simulink model "step1"  (R2026a)
settings: Solver=VariableStepAuto
undefined symbols (not defined in the file): F_drive, m
settings Model: Creator=manoj  LastModifiedBy=manoj

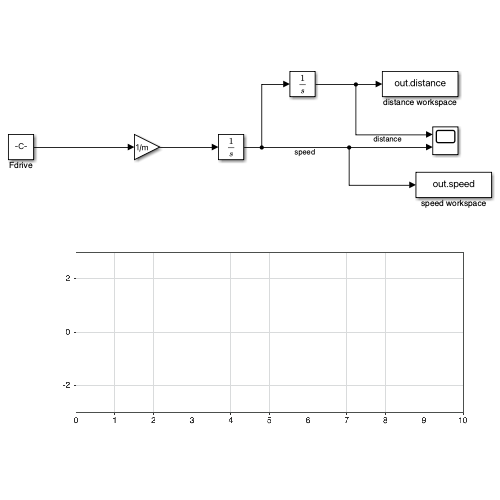
[thumbnail: Simulink's stored preview of the top-level diagram]
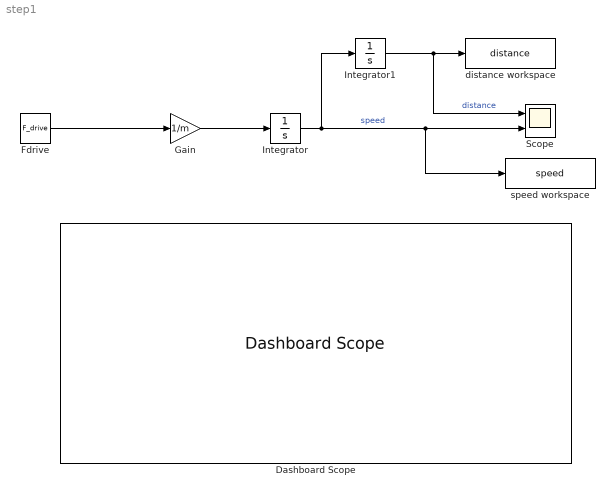
== system step1 ==
  Dashboard Scope : DashboardScope  FontColor=[0.0, 0.0, 0.0]
  Fdrive : Constant  Value=F_drive
  Gain : Gain  Gain=1/m
  Integrator : Integrator
  Integrator1 : Integrator
  Scope : Scope  NumInputPorts=2
      settings: ActiveDisplayYMinimum=-1  ActiveDisplayYMaximum=1
  distance workspace : ToWorkspace  VariableName=distance  SaveFormat=Structure With Time  SampleTime=-1
  speed workspace : ToWorkspace  VariableName=speed  SaveFormat=Structure With Time  SampleTime=-1
  wires:
  Integrator/1 -> Integrator1/1, speed workspace/1, Scope/2  "speed"
  Gain/1 -> Integrator/1
  Fdrive/1 -> Gain/1
  Integrator1/1 -> distance workspace/1, Scope/1  "distance"
